simulink model "DFK_mdl"  (R2013a)
settings: Solver=ode45  StartTime=0.0  StopTime=inf  RelTol=1e-3
undefined symbols (not defined in the file or in its folder): HIK, ToSimulink_Y_Signals2VRML
libraries: simulink x5, vrlib x1
settings Model: Creator=Jose Angel Rangel  LastModifiedBy=Jose Angel Rangel

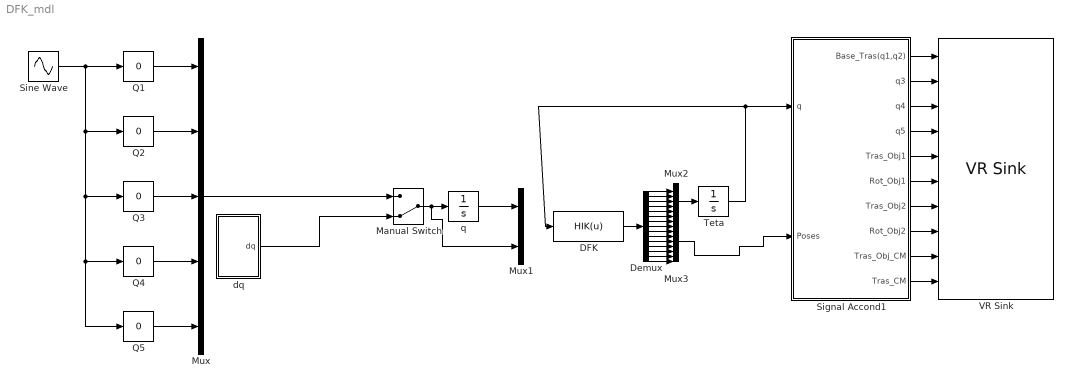
== system DFK_mdl ==
  DFK : MATLABFcn  MATLABFcn=HIK(u)
  Demux : Demux  Outputs=15
  Manual Switch : ManualSwitch  CurrentSetting=0
  Mux : Mux  Inputs=5
  Mux1 : Mux  Inputs=2
  Mux2 : Mux  Inputs=5
  Mux3 : Mux  Inputs=10
  Q{1..5} (5 alike) : simulink/Math Operations/Slider Gain  low=-5  gain=0  high=5
  Signal Accond1 : Subsystem
  Sine Wave : Sin  SampleTime=0
  Teta : Integrator
  VR Sink : vrlib/VR Sink  InstantiateOnLoad=on  SampleTime=0.1  ViewEnable=on  RemoteChange=off  RemoteView=off  FieldsWritten=Base_Tras.translation.3.1.1.double#Base_Rot.rotation.4.1.1.double#Q4.rotation.4.1.1.double#Q5.rotation.4.1.1.double#Obj_RH.translation.3.1.1.double#Rot_Obj_RH.rotation.4.1.1.double#Obj_LH.translation.3.1.1.double#Rot_Obj_LH.rotation.4.1.1.double#Obj_CM.translation.3.1.1.double#Actual_CM.translation.3.1.1.double  WorldFileName=Simpley.wrl  AutoView=on  VideoDimensions=[]  AllowVariableSize=off  FigureProperties="{'Position', 'Name', 'Viewpoint', 'CameraBound', 'CameraDirection', 'CameraPosition', 'CameraUpVector', 'ZoomFactor', 'Antialiasing', 'Headlight', 'Lighting', 'NavPanel', 'StatusBar', 'ToolBar', 'Textures', 'Transparency', 'Triad', 'Wireframe', 'NavZones', 'NavMode', 'NavSpeed', 'CaptureFileFormat', 'CaptureFileName', 'Record2DCompressMethod', 'Record2DCompressQuality', 'Record2D', 'Record2DFileName', 'Record2DFPS'; [5.0000000000000000e+00   9.2000000000000000e+01   5.7600000000000000e+02   3.8000000000000000e+02], '', '_untitled_1', 'on', [0.0000000000000000e+00   0.0000000000000000e+00  -1.0000000000000000e+00], [0.0000000000000000e+00   0.0000000000000000e+00   2.0000000000000000e+01], [0.0000000000000000e+00   1.0000000000000000e+00   0.0000000000000000e+00], [1.0000000000000000e+00], 'on', 'on', 'on', 'halfbar', 'on', 'on', 'on', 'on', 'none', 'off', 'off', 'fly', 'normal', 'tif', '%f_anim_%n.tif', 'auto', [7.5000000000000000e+01], 'off', '%f_anim_%n.avi', [1.5000000000000000e+01]}"
  dq : Subsystem
  q : Integrator
  wires:
  Sine Wave/1 -> Q2/1, Q3/1, Q4/1, Q5/1, Q1/1
  Q1/1 -> Mux/1
  Q2/1 -> Mux/2
  Q3/1 -> Mux/3
  Q4/1 -> Mux/4
  Q5/1 -> Mux/5
  DFK/1 -> Demux/1
  q/1 -> Mux1/1
  Mux2/1 -> Teta/1
  Mux3/1 -> Signal Accond1/2(Poses)
  Manual Switch/1 -> Mux1/2, q/1
  Mux/1 -> Manual Switch/1
  dq/1(dq) -> Manual Switch/2
  Signal Accond1/10(Tras_CM) -> VR Sink/10
  Signal Accond1/9(Tras_Obj_CM) -> VR Sink/9
  Signal Accond1/8(Rot_Obj2) -> VR Sink/8
  Signal Accond1/7(Tras_Obj2) -> VR Sink/7
  Signal Accond1/6(Rot_Obj1) -> VR Sink/6
  Signal Accond1/5(Tras_Obj1) -> VR Sink/5
  Signal Accond1/4(q5) -> VR Sink/4
  Signal Accond1/3(q4) -> VR Sink/3
  Signal Accond1/2(q3) -> VR Sink/2
  Signal Accond1/1(Base_Tras(q1,q2)) -> VR Sink/1
  Demux/1 -> Mux2/1
  Demux/2 -> Mux2/2
  Demux/3 -> Mux2/3
  Demux/4 -> Mux2/4
  Demux/5 -> Mux2/5
  Demux/6 -> Mux3/1
  Demux/8 -> Mux3/3
  Demux/7 -> Mux3/2
  Demux/9 -> Mux3/4
  Demux/10 -> Mux3/5
  Demux/11 -> Mux3/6
  Demux/12 -> Mux3/7
  Demux/14 -> Mux3/9
  Demux/13 -> Mux3/8
  Demux/15 -> Mux3/10
  Teta/1 -> Signal Accond1/1(q), DFK/1

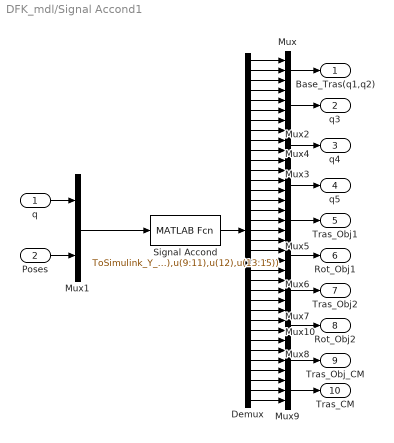
== system DFK_mdl/Signal Accond1 ==
  q : Inport
  Poses : Inport  Port=2
  Demux : Demux  Outputs=35
  Mux{,5,7,9..10} (5 alike) : Mux  Inputs=3
  Mux1 : Mux  Inputs=2
  Mux{2..4,6,8} (5 alike) : Mux
  Signal Accond : MATLABFcn  MATLABFcn=ToSimulink_Y_Signals2VRML(u(1:5),u(6:8),u(9:11),u(12),u(13:15))  OutputDimensions=35
  Base_Tras(q1,q2) : Outport
  q3 : Outport  Port=2
  q4 : Outport  Port=3
  q5 : Outport  Port=4
  Tras_Obj1 : Outport  Port=5
  Rot_Obj1 : Outport  Port=6
  Tras_Obj2 : Outport  Port=7
  Rot_Obj2 : Outport  Port=8
  Tras_Obj_CM : Outport  Port=9
  Tras_CM : Outport  Port=10
  wires:
  q/1 -> Mux1/1
  Poses/1 -> Mux1/2
  Mux1/1 -> Signal Accond/1
  Signal Accond/1 -> Demux/1
  Mux/1 -> Base_Tras(q1,q2)/1
  Mux2/1 -> q3/1
  Mux3/1 -> q4/1
  Mux4/1 -> q5/1
  Mux5/1 -> Tras_Obj1/1
  Mux6/1 -> Rot_Obj1/1
  Mux7/1 -> Tras_Obj2/1
  Mux8/1 -> Rot_Obj2/1
  Mux10/1 -> Tras_Obj_CM/1
  Demux/28 -> Mux8/3
  Demux/24 -> Mux7/2
  Demux/25 -> Mux7/3
  Demux/4 -> Mux2/1
  Demux/11 -> Mux3/4
  Demux/9 -> Mux3/2
  Demux/27 -> Mux8/2
  Demux/14 -> Mux4/3
  Demux/7 -> Mux2/4
  Demux/5 -> Mux2/2
  Demux/13 -> Mux4/2
  Demux/1 -> Mux/1
  Demux/19 -> Mux6/1
  Demux/6 -> Mux2/3
  Demux/3 -> Mux/3
  Demux/26 -> Mux8/1
  Demux/20 -> Mux6/2
  Demux/16 -> Mux5/1
  Demux/15 -> Mux4/4
  Demux/2 -> Mux/2
  Demux/21 -> Mux6/3
  Demux/23 -> Mux7/1
  Demux/10 -> Mux3/3
  Demux/12 -> Mux4/1
  Demux/22 -> Mux6/4
  Demux/18 -> Mux5/3
  Demux/17 -> Mux5/2
  Demux/29 -> Mux8/4
  Demux/8 -> Mux3/1
  Demux/32 -> Mux10/3
  Demux/31 -> Mux10/2
  Demux/30 -> Mux10/1
  Mux9/1 -> Tras_CM/1
  Demux/35 -> Mux9/3
  Demux/34 -> Mux9/2
  Demux/33 -> Mux9/1

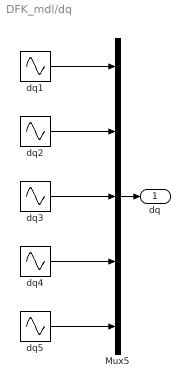
== system DFK_mdl/dq ==
  Mux5 : Mux  Inputs=5
  dq1 : Sin  Amplitude=2*pi  SampleTime=0
  dq2 : Sin  Amplitude=pi  Frequency=0.8  SampleTime=0
  dq3 : Sin  Amplitude=3*pi/4  Frequency=0.5  SampleTime=0
  dq4 : Sin  Amplitude=5  Frequency=2  SampleTime=0
  dq5 : Sin  Amplitude=5  Frequency=0.1  SampleTime=0
  dq : Outport
  wires:
  dq1/1 -> Mux5/1
  dq2/1 -> Mux5/2
  dq5/1 -> Mux5/5
  dq4/1 -> Mux5/4
  dq3/1 -> Mux5/3
  Mux5/1 -> dq/1
